simulink model "TreciZad"  (R2016b)
settings: Solver=VariableStepAuto  StartTime=0.0  StopTime=800  RelTol=1e-3
libraries: simulink x3
settings Model: Creator=Luka  LastModifiedBy=Luka

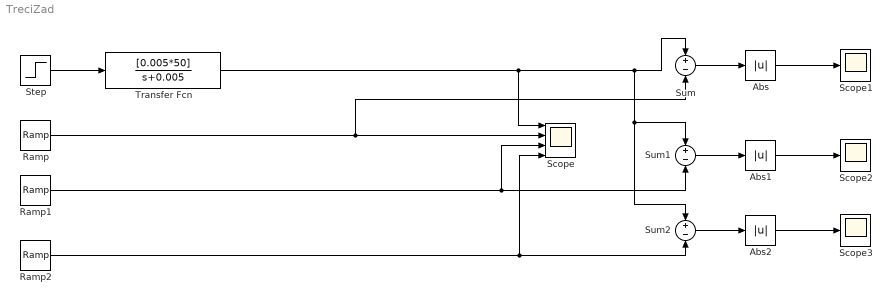
== system TreciZad ==
  Abs : Abs
  Abs1 : Abs
  Abs2 : Abs
  Ramp : simulink/Sources/Ramp  slope=0.0613  start=0  X0=0
  Ramp1 : simulink/Sources/Ramp  slope=0.0426  start=0  X0=20.696
  Ramp2 : simulink/Sources/Ramp  slope=0.092  start=0  X0=13.2
  Scope : Scope  NumInputPorts=4
  Scope1 : Scope
  Scope2 : Scope
  Scope3 : Scope
  Step : Step  Time=0  SampleTime=0
  Sum : Sum  Inputs=+-
  Sum1 : Sum  Inputs=+-
  Sum2 : Sum  Inputs=+-
  Transfer Fcn : TransferFcn  Numerator=[0.005*50]  Denominator=[1 0.005]
  wires:
  Step/1 -> Transfer Fcn/1
  Transfer Fcn/1 -> Sum1/1, Sum2/1, Sum/1, Scope/1
  Ramp/1 -> Sum/2, Scope/2
  Ramp1/1 -> Sum1/2, Scope/3
  Ramp2/1 -> Sum2/2, Scope/4
  Abs/1 -> Scope1/1
  Abs1/1 -> Scope2/1
  Abs2/1 -> Scope3/1
  Sum2/1 -> Abs2/1
  Sum1/1 -> Abs1/1
  Sum/1 -> Abs/1
